simulink model "pendulum"  (R2015b)
settings: Solver=ode45  StartTime=0.0  StopTime=10.0  MaxStep=0.01  RelTol=1e-3
values from neighbouring files (symbols this model uses):
  d = 0.2    [init_pendulum.m]
  g = 9.81    [init_pendulum.m]
  l = 1.5    [init_pendulum.m]
  m = 0.5    [init_pendulum.m]
  phi_0 = 178 / 180 * pi    (= 3.10668606855)    [init_pendulum.m]
  phi_dot_0 = 0    [init_pendulum.m]
settings Model: Creator=Goettlicher  LastModifiedBy=Goettlicher
settings DebuggingCC: SignalLabelMismatchMsg=error  BusObjectLabelMismatch=error  RootOutportRequireBusObject=error

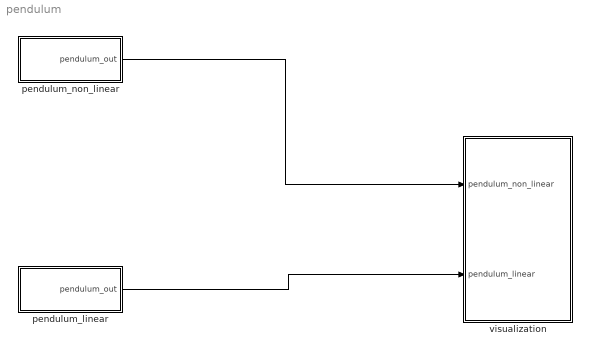
== system pendulum ==
  pendulum_linear : Subsystem
  pendulum_non_linear : Subsystem
  visualization : Subsystem
  wires:
  pendulum_non_linear/1(pendulum_out) -> visualization/1(pendulum_non_linear)
  pendulum_linear/1(pendulum_out) -> visualization/2(pendulum_linear)

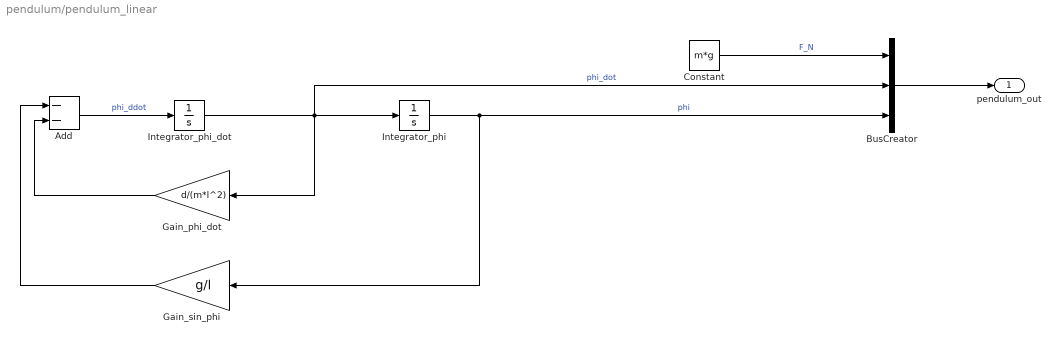
== system pendulum/pendulum_linear ==
  Add : Sum  Inputs=--
  BusCreator : BusCreator  Inputs=3  OutDataTypeStr=Bus: pendulum_bus
  Constant : Constant  Value=m*g
  Gain_phi_dot : Gain  Gain=d/(m*l^2)
  Gain_sin_phi : Gain  Gain=g/l
  Integrator_phi : Integrator  InitialCondition=phi_0
  Integrator_phi_dot : Integrator  InitialCondition=phi_dot_0
  pendulum_out : Outport  OutDataTypeStr=Bus: pendulum_bus
  wires:
  Constant/1 -> BusCreator/1  "F_N"
  BusCreator/1 -> pendulum_out/1
  Gain_sin_phi/1 -> Add/1
  Gain_phi_dot/1 -> Add/2
  Add/1 -> Integrator_phi_dot/1  "phi_ddot"
  Integrator_phi/1 -> Gain_sin_phi/1, BusCreator/3  "phi"
  Integrator_phi_dot/1 -> Integrator_phi/1, Gain_phi_dot/1, BusCreator/2  "phi_dot"

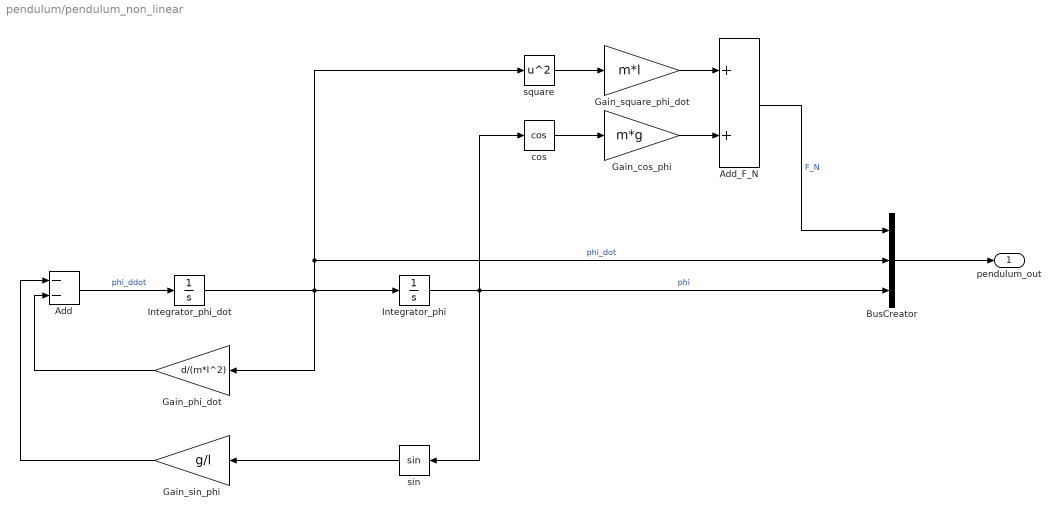
== system pendulum/pendulum_non_linear ==
  Add : Sum  Inputs=--
  Add_F_N : Sum
  BusCreator : BusCreator  Inputs=3  OutDataTypeStr=Bus: pendulum_bus
  Gain_cos_phi : Gain  Gain=m*g
  Gain_phi_dot : Gain  Gain=d/(m*l^2)
  Gain_sin_phi : Gain  Gain=g/l
  Gain_square_phi_dot : Gain  Gain=m*l
  Integrator_phi : Integrator  InitialCondition=phi_0
  Integrator_phi_dot : Integrator  InitialCondition=phi_dot_0
  cos : Trigonometry  Operator=cos
  sin : Trigonometry
  square : Math  Operator=square  SaturateOnIntegerOverflow=on
  pendulum_out : Outport  OutDataTypeStr=Bus: pendulum_bus
  wires:
  Integrator_phi_dot/1 -> square/1, BusCreator/2, Gain_phi_dot/1, Integrator_phi/1  "phi_dot"
  Integrator_phi/1 -> cos/1, sin/1, BusCreator/3  "phi"
  Add/1 -> Integrator_phi_dot/1  "phi_ddot"
  sin/1 -> Gain_sin_phi/1
  Gain_phi_dot/1 -> Add/2
  Gain_sin_phi/1 -> Add/1
  BusCreator/1 -> pendulum_out/1
  Add_F_N/1 -> BusCreator/1  "F_N"
  cos/1 -> Gain_cos_phi/1
  square/1 -> Gain_square_phi_dot/1
  Gain_square_phi_dot/1 -> Add_F_N/1
  Gain_cos_phi/1 -> Add_F_N/2

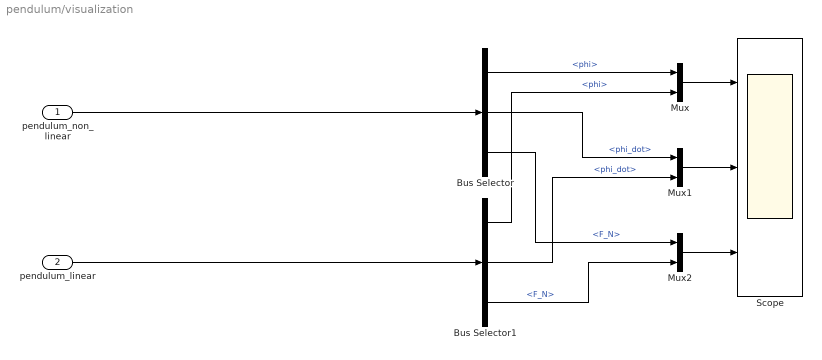
== system pendulum/visualization ==
  pendulum_non_linear : Inport  OutDataTypeStr=Bus: pendulum_bus
  pendulum_linear : Inport  Port=2  OutDataTypeStr=Bus: pendulum_bus
  Bus Selector : BusSelector  OutputSignals=phi,phi_dot,F_N
  Bus Selector1 : BusSelector  OutputSignals=phi,phi_dot,F_N
  Mux : Mux  Inputs=2
  Mux1 : Mux  Inputs=2
  Mux2 : Mux  Inputs=2
  Scope : Scope  NumInputPorts=3
  wires:
  Mux/1 -> Scope/1
  Mux1/1 -> Scope/2
  Mux2/1 -> Scope/3
  pendulum_non_linear/1 -> Bus Selector/1
  Bus Selector/1 -> Mux/1  "<phi>"
  Bus Selector/2 -> Mux1/1  "<phi_dot>"
  Bus Selector/3 -> Mux2/1  "<F_N>"
  pendulum_linear/1 -> Bus Selector1/1
  Bus Selector1/1 -> Mux/2  "<phi>"
  Bus Selector1/2 -> Mux1/2  "<phi_dot>"
  Bus Selector1/3 -> Mux2/2  "<F_N>"
